simulink model "A2"  (R2024a)
settings: Solver=ode4  StartTime=0.0  StopTime=20  RelTol=1e-3
settings Model: Creator=Flipper  LastModifiedBy=Flipper

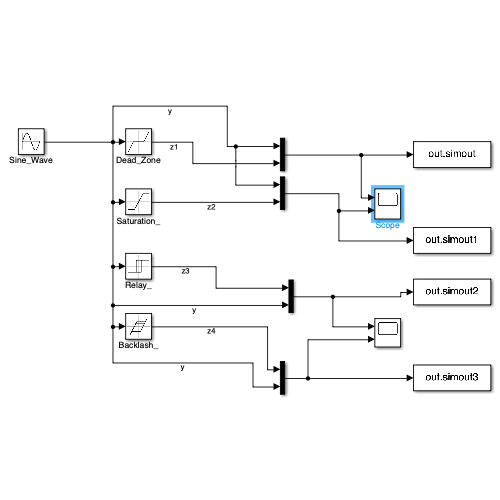
[thumbnail: Simulink's stored preview of the top-level diagram]
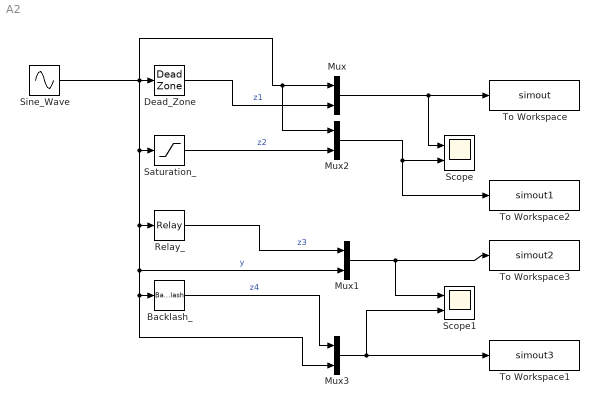
== system A2 ==
  Backlash_ : Backlash
  Dead_Zone : DeadZone
  Mux{,1..3} (4 alike) : Mux  Inputs=2
  Relay_ : Relay  OnOutputValue=0.5  OffOutputValue=-0.5
  Saturation_ : Saturate
  Scope : Scope  NumInputPorts=2
  Scope1 : Scope  NumInputPorts=2
  Sine_Wave : Sin  Amplitude=2  Frequency=1/2  SampleTime=0
  To Workspace : ToWorkspace  VariableName=simout  SaveFormat=Timeseries  SampleTime=-1
  To Workspace1 : ToWorkspace  VariableName=simout3  SaveFormat=Timeseries  SampleTime=-1
  To Workspace2 : ToWorkspace  VariableName=simout1  SaveFormat=Timeseries  SampleTime=-1
  To Workspace3 : ToWorkspace  VariableName=simout2  SaveFormat=Timeseries  SampleTime=-1
  wires:
  Sine_Wave/1 -> Mux1/2, Mux3/2, Backlash_/1, Relay_/1, Saturation_/1, Mux2/1, Mux/1, Dead_Zone/1  "y"
  Backlash_/1 -> Mux3/1  "z4"
  Relay_/1 -> Mux1/1  "z3"
  Saturation_/1 -> Mux2/2  "z2"
  Dead_Zone/1 -> Mux/2  "z1"
  Mux/1 -> Scope/1, To Workspace/1
  Mux1/1 -> Scope1/1, To Workspace3/1
  Mux2/1 -> To Workspace2/1, Scope/2
  Mux3/1 -> Scope1/2, To Workspace1/1
